simulink model "MSFartoystyring22"  (R2017b)
settings: Solver=ode45  StartTime=tstart  StopTime=tstop  RelTol=1e-3  EnableMultiTasking=on
values from neighbouring files (symbols this model uses):
  c = 1    [run22.m]
  p0 = [1500 500]    [run22.m]
  psi0 = 50*deg2rad    (= 0.872664625997)    [run22.m]
  r0 = 0    [run22.m]
  tsamp = 10    [run22.m]
  u_r_0 = v0(1)    [run22.m]
  v0 = [6.63 0]'    [run22.m]
undefined symbols (not defined in the file or in its folder): d1, d2, K, Kd_heading, Ki_heading, Ki_speed, Kp_heading, Kp_speed, m, msfartoystyring, omega_c, omega_n, T, WP, zeta_c
settings Model: ExtModeAutoUpdateStatusClock=off  Creator=christh  LastModifiedBy=henningward
settings SolverCC: ZeroCrossAlgorithm=Adaptive
settings DataIOCC: LimitDataPoints=on  SaveFormat=Array  SignalLoggingSaveFormat=ModelDataLogs
settings OptimizationCC: ExpressionDepthLimit=2147483647  InitFltsAndDblsToZero=on  LifeSpan=inf
settings DebuggingCC: UnderspecifiedInitializationDetection=Classic  MergeDetectMultiDrivingBlocksExec=none  IgnoredZcDiagnostic=none  SolverPrmCheckMsg=warning  FcnCallInpInsideContextMsg=warning  StateNameClashWarn=warning  SFUnexpectedBacktrackingDiag=warning  SFNoUnconditionalDefaultTransitionDiag=warning  SFExecutionAtInitializationDiag=none
settings HardwareCC: ProdBitPerPointer=32  ProdBitPerSizeT=32  ProdBitPerPtrDiffT=32  ProdLargestAtomicFloat=None  ProdIntDivRoundTo=Undefined  ProdEndianess=Unspecified  ProdWordSize=32  ProdHWDeviceType=32-bit Generic
settings ModelReferenceCC: PropagateSignalLabelsOutOfModel=off
settings CodeAppCC: StateflowObjectComments=on
settings GRTTargetCC: TargetLangStandard=C89/C90 (ANSI)  GeneratePreprocessorConditionals=Disable all  CombineOutputUpdateFcns=off  GRTInterface=on
settings ConfigComp: CovMetricSettings=dw  CovHtmlReporting=on  CovSaveCumulativeToWorkspaceVar=on  CovSaveSingleToWorkspaceVar=on  CovExternalEMLEnable=off

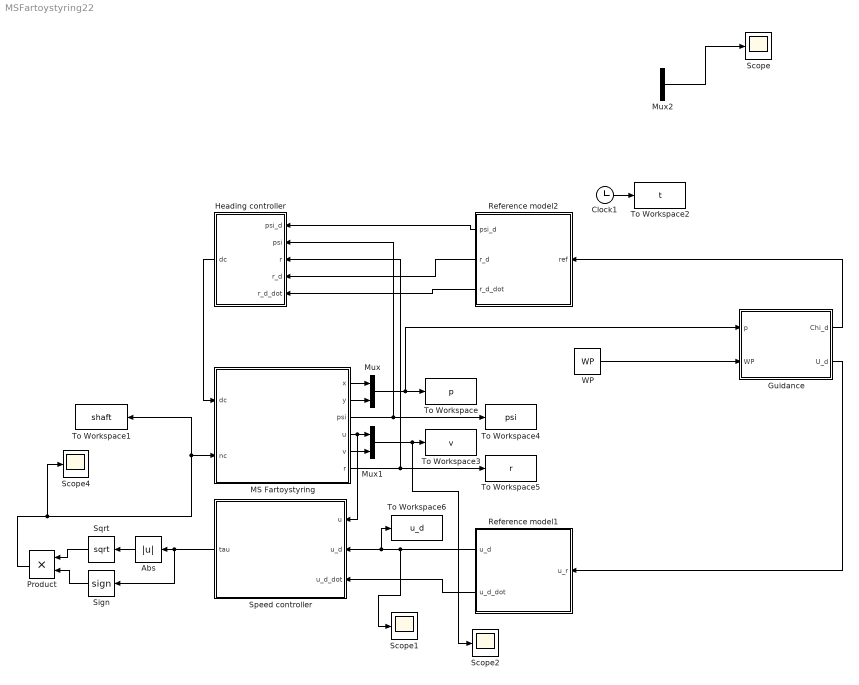
== system MSFartoystyring22 ==
  Abs : Abs
  Clock1 : Clock
  "Guidance " : Subsystem
  Heading controller : Subsystem
  MS Fartoystyring : Subsystem  mask(MS Fartoystyring for Assignment 3 G&C){x0=p0(1), y0=p0(2), u0=v0(1), v0=v0(2), psi0=psi0, r0=r0, c=c}
      mask prompts: x0 "x(t0) (m)"; y0 "y(t0) (m)"; u0 "u(t0) (m/s)"; v0 "v(t0) (m/s)"; psi0 "psi(t0) (rad)"; r0 "r(t0) (rad/s)"; c "current (0 or 1)"
      mask help:
      | Block corresponding to Figure 1 in the assignment text. Gives the response of the ship.
      |
      | The design speed of MS Fartoystyring is u=8.23 m/s.
      |
      | Input:
      | dc: commanded rudder (rad), dmax=25*pi/180
      | nc: commanded shaft speed (rad/s), nmax=85*2*pi/60
      |
      | Output:
      | x: north pos (m)
      | y: east pos (m)
      | u: surge (m/s)
      | v: sway (m/s)
      | psi: heading (rad)
      | r: yaw (rad/s)
      mask Help: Comments, bugs and help requests can be directed to the TA. Email on course website.
  Mux : Mux  Inputs=2
  Mux1 : Mux  Inputs=2
  Mux2 : Mux  Inputs=2
  Product : Product
  Reference model1 : Subsystem
  Reference model2 : Subsystem
  Scope{,1..2,4} (4 alike) : Scope
  Sign : Signum
  Speed controller : Subsystem
  Sqrt : Sqrt  SaturateOnIntegerOverflow=on
  To Workspace : ToWorkspace  VariableName=p  SampleTime=tsamp
  To Workspace1 : ToWorkspace  VariableName=shaft  SampleTime=tsamp
  To Workspace2 : ToWorkspace  VariableName=t  SampleTime=tsamp
  To Workspace3 : ToWorkspace  VariableName=v  SampleTime=tsamp
  To Workspace4 : ToWorkspace  VariableName=psi  SampleTime=tsamp
  To Workspace5 : ToWorkspace  VariableName=r  SampleTime=tsamp
  To Workspace6 : ToWorkspace  VariableName=u_d  SampleTime=tsamp
  WP : Constant  Value=WP
  wires:
  MS Fartoystyring/1(x) -> Mux/1
  MS Fartoystyring/2(y) -> Mux/2
  MS Fartoystyring/4(u) -> Speed controller/1("u "), Mux1/1
  MS Fartoystyring/5(v) -> Mux1/2
  Mux/1 -> "Guidance "/1(p), To Workspace/1
  Clock1/1 -> To Workspace2/1
  Speed controller/1("tau ") -> Sign/1, Abs/1
  Abs/1 -> Sqrt/1
  Sign/1 -> Product/2
  Sqrt/1 -> Product/1
  Product/1 -> Scope4/1, To Workspace1/1, MS Fartoystyring/2(nc)
  Reference model1/1(u_d) -> Scope1/1, To Workspace6/1, Speed controller/2(u_d)
  Reference model1/2(u_d_dot) -> Speed controller/3(u_d_dot)
  WP/1 -> "Guidance "/2(WP)
  Reference model2/2(r_d) -> Heading controller/4(r_d)
  MS Fartoystyring/6(r) -> Heading controller/3(r), To Workspace5/1
  MS Fartoystyring/3(psi) -> Heading controller/2(psi), To Workspace4/1
  Reference model2/3("r_d_dot ") -> Heading controller/5("r_d_dot ")
  Mux1/1 -> Scope2/1, To Workspace3/1
  Heading controller/1(dc) -> MS Fartoystyring/1(dc)
  Reference model2/1(psi_d) -> Heading controller/1(psi_d)
  Mux2/1 -> Scope/1
  "Guidance "/1("Chi_d ") -> Reference model2/1(ref)
  "Guidance "/2(U_d) -> Reference model1/1(u_r)

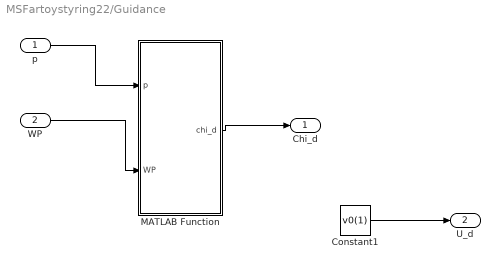
== system MSFartoystyring22/Guidance  ==
  p : Inport
  WP : Inport  Port=2
  Constant1 : Constant  Value=v0(1)
  MATLAB Function : MATLAB Function  TreatAsAtomicUnit=on
  "Chi_d " : Outport
  U_d : Outport  Port=2
  wires:
  p/1 -> MATLAB Function/1(p)
  WP/1 -> MATLAB Function/2(WP)
  Constant1/1 -> U_d/1
  MATLAB Function/1(chi_d) -> "Chi_d "/1

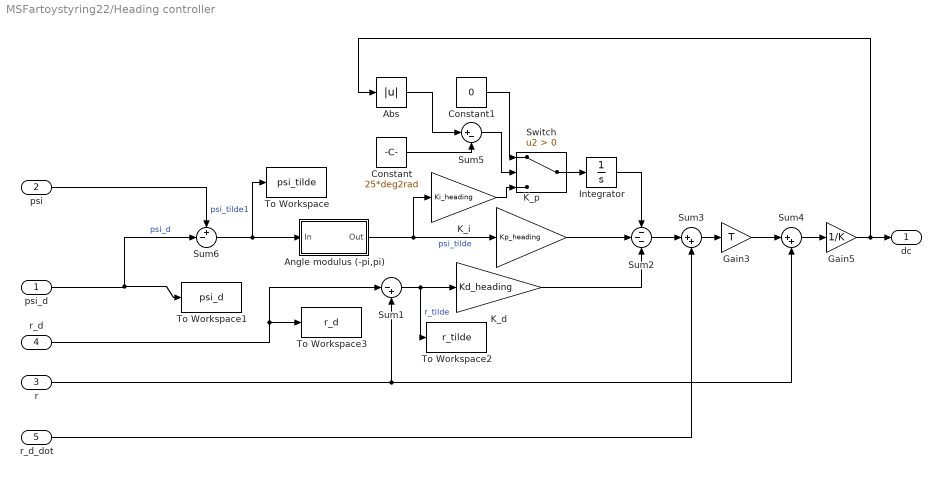
== system MSFartoystyring22/Heading controller ==
  psi_d : Inport
  psi : Inport  Port=2
  r : Inport  Port=3
  r_d : Inport  Port=4
  "r_d_dot " : Inport  Port=5
  Abs : Abs
  Angle modulus (-pi,pi) : Subsystem
  Constant : Constant  Value=25*deg2rad
  Constant1 : Constant  Value=0
  Gain3 : Gain  Gain=T
  Gain5 : Gain  Gain=1/K
  Integrator : Integrator  LimitOutput=on  UpperSaturationLimit=deg2rad*25*abs(K)/T  LowerSaturationLimit=-deg2rad*25*abs(K)/T
  K_d : Gain  Gain=Kd_heading
  K_i : Gain  Gain=Ki_heading
  K_p : Gain  Gain=Kp_heading
  Sum1 : Sum  Inputs=|-+
  Sum2 : Sum  Inputs=---
  Sum3 : Sum  Inputs=|++
  Sum4 : Sum  Inputs=|++
  Sum5 : Sum  Inputs=|+-
  Sum6 : Sum  Inputs=+-|
  Switch : Switch  Criteria=u2 > Threshold
  To Workspace : ToWorkspace  VariableName=psi_tilde  SampleTime=tsamp
  To Workspace1 : ToWorkspace  VariableName=psi_d  SampleTime=tsamp
  To Workspace2 : ToWorkspace  VariableName=r_tilde  SampleTime=tsamp
  To Workspace3 : ToWorkspace  VariableName=r_d  SampleTime=tsamp
  dc : Outport
  wires:
  Sum1/1 -> To Workspace2/1, K_d/1  "r_tilde"
  Angle modulus (-pi,pi)/1(Out) -> K_p/1, K_i/1  "psi_tilde"
  K_p/1 -> Sum2/2
  Sum2/1 -> Sum3/1
  K_d/1 -> Sum2/3
  Sum3/1 -> Gain3/1
  Gain3/1 -> Sum4/1
  r/1 -> Sum4/2, Sum1/2
  Gain5/1 -> Abs/1, dc/1
  Sum4/1 -> Gain5/1
  Integrator/1 -> Sum2/1
  Abs/1 -> Sum5/1
  Sum5/1 -> Switch/2
  Constant/1 -> Sum5/2
  Constant1/1 -> Switch/1
  K_i/1 -> Switch/3
  Switch/1 -> Integrator/1
  psi_d/1 -> To Workspace1/1, Sum6/2  "psi_d"
  Sum6/1 -> To Workspace/1, Angle modulus (-pi,pi)/1(In)  "psi_tilde1"
  psi/1 -> Sum6/1
  "r_d_dot "/1 -> Sum3/2
  r_d/1 -> To Workspace3/1, Sum1/1

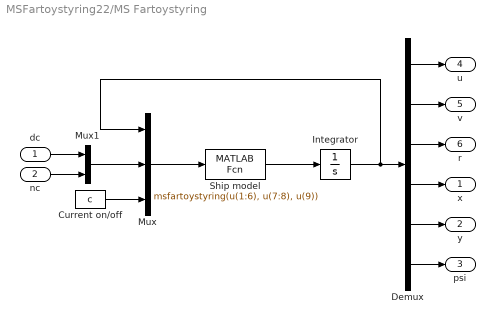
== system MSFartoystyring22/MS Fartoystyring ==
  dc : Inport
  nc : Inport  Port=2
  Current on/off : Constant  Value=c
  Demux : Demux  Outputs=6
  Integrator : Integrator  InitialCondition=[u0 v0 r0 x0 y0 psi0]'
  Mux : Mux  Inputs=3
  Mux1 : Mux  Inputs=2
  Ship model : MATLABFcn  MATLABFcn=msfartoystyring(u(1:6), u(7:8), u(9))  OutputDimensions=6
  x : Outport
  y : Outport  Port=2
  psi : Outport  Port=3
  u : Outport  Port=4
  v : Outport  Port=5
  r : Outport  Port=6
  wires:
  Integrator/1 -> Mux/1, Demux/1
  Mux1/1 -> Mux/2
  dc/1 -> Mux1/1
  nc/1 -> Mux1/2
  Demux/1 -> u/1
  Demux/2 -> v/1
  Demux/3 -> r/1
  Demux/4 -> x/1
  Demux/5 -> y/1
  Demux/6 -> psi/1
  Current on/off/1 -> Mux/3
  Ship model/1 -> Integrator/1
  Mux/1 -> Ship model/1

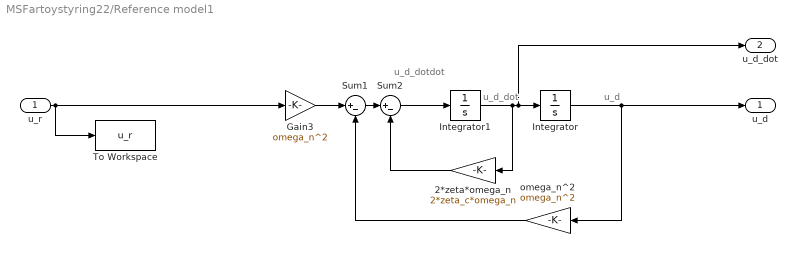
== system MSFartoystyring22/Reference model1 ==
  note: u_d
  note: u_d_dot
  note: u_d_dotdot
  u_r : Inport
  2*zeta*omega_n : Gain  Gain=2*zeta_c*omega_n
  Gain3 : Gain  Gain=omega_n^2
  Integrator : Integrator  InitialCondition=u_r_0
  Integrator1 : Integrator
  Sum1 : Sum  Inputs=|+-
  Sum2 : Sum  Inputs=|+-
  To Workspace : ToWorkspace  VariableName=u_r  SampleTime=-1
  omega_n^2 : Gain  Gain=omega_n^2
  u_d : Outport
  u_d_dot : Outport  Port=2
  wires:
  Integrator1/1 -> 2*zeta*omega_n/1, Integrator/1, u_d_dot/1
  2*zeta*omega_n/1 -> Sum2/2
  Sum1/1 -> Sum2/1
  omega_n^2/1 -> Sum1/2
  Gain3/1 -> Sum1/1
  Sum2/1 -> Integrator1/1
  Integrator/1 -> omega_n^2/1, u_d/1
  u_r/1 -> To Workspace/1, Gain3/1

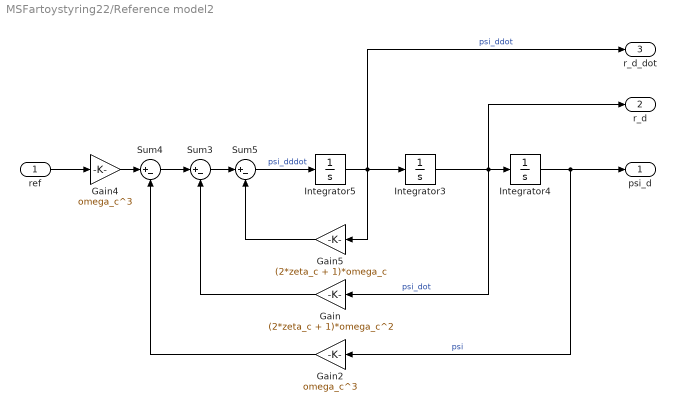
== system MSFartoystyring22/Reference model2 ==
  ref : Inport
  Gain : Gain  Gain=(2*zeta_c + 1)*omega_c^2
  Gain2 : Gain  Gain=omega_c^3
  Gain4 : Gain  Gain=omega_c^3
  Gain5 : Gain  Gain=(2*zeta_c + 1)*omega_c
  Integrator3 : Integrator
  Integrator4 : Integrator  InitialCondition=psi0
  Integrator5 : Integrator
  Sum3 : Sum  Inputs=|+-
  Sum4 : Sum  Inputs=|+-
  Sum5 : Sum  Inputs=|+-
  psi_d : Outport
  r_d : Outport  Port=2
  "r_d_dot " : Outport  Port=3
  wires:
  Integrator3/1 -> r_d/1, Gain/1, Integrator4/1  "psi_dot"
  Gain/1 -> Sum3/2
  ref/1 -> Gain4/1
  Integrator4/1 -> psi_d/1, Gain2/1  "psi"
  Sum4/1 -> Sum3/1
  Gain4/1 -> Sum4/1
  Sum3/1 -> Sum5/1
  Gain5/1 -> Sum5/2
  Sum5/1 -> Integrator5/1  "psi_dddot"
  Gain2/1 -> Sum4/2
  Integrator5/1 -> Gain5/1, "r_d_dot "/1, Integrator3/1  "psi_ddot"

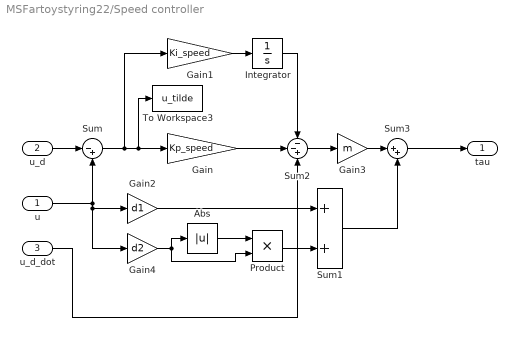
== system MSFartoystyring22/Speed controller ==
  "u " : Inport
  u_d : Inport  Port=2
  u_d_dot : Inport  Port=3
  Abs : Abs
  Gain : Gain  Gain=Kp_speed
  Gain1 : Gain  Gain=Ki_speed
  Gain2 : Gain  Gain=d1
  Gain3 : Gain  Gain=m
  Gain4 : Gain  Gain=d2
  Integrator : Integrator
  Product : Product
  Sum : Sum  Inputs=|-+
  Sum1 : Sum
  Sum2 : Sum  Inputs=--+
  Sum3 : Sum  Inputs=|++
  To Workspace3 : ToWorkspace  VariableName=u_tilde  SampleTime=tsamp
  "tau " : Outport
  wires:
  Integrator/1 -> Sum2/1
  Gain/1 -> Sum2/2
  Sum2/1 -> Gain3/1
  Gain3/1 -> Sum3/1
  u_d_dot/1 -> Sum2/3
  Sum/1 -> To Workspace3/1, Gain/1, Gain1/1
  Gain1/1 -> Integrator/1
  u_d/1 -> Sum/1
  "u "/1 -> Gain4/1, Gain2/1, Sum/2
  Abs/1 -> Product/1
  Gain4/1 -> Abs/1, Product/2
  Gain2/1 -> Sum1/1
  Product/1 -> Sum1/2
  Sum1/1 -> Sum3/2
  Sum3/1 -> "tau "/1

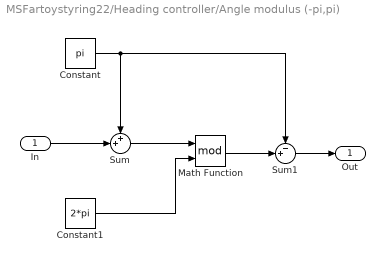
== system MSFartoystyring22/Heading controller/Angle modulus (-pi,pi) ==
  In : Inport
  Constant : Constant  Value=pi
  Constant1 : Constant  Value=2*pi
  Math Function : Math  Operator=mod  SaturateOnIntegerOverflow=on
  Sum : Sum  Inputs=++|
  Sum1 : Sum  Inputs=-+|
  Out : Outport
  wires:
  Math Function/1 -> Sum1/2
  Sum/1 -> Math Function/1
  Constant/1 -> Sum1/1, Sum/1
  In/1 -> Sum/2
  Sum1/1 -> Out/1
  Constant1/1 -> Math Function/2

== matlab function MSFartoystyring22/Guidance /MATLAB Function ==
  settings: updateMethod=DISCRETE  sampleTime=tsamp
  data: p input; chi_d output; WP input
function chi_d = fcn(p, WP)

    %number of waypoints
    N = length(WP);

    % waypoint iteration
    persistent k;
    
    %waypoint iteration
    if (isempty(k))
        k = 1;
    end
    
    %reference waypoint
    xk_ref = WP(1, k);
    yk_ref = WP(2, k);
    
    %next waypoint
    xk_target = WP(1, k+1);
    yk_target = WP(2, k+1);
    
    
    if k ~= 6 && k ~= 1
        %calculating optimal turningradius
        lastWP = [WP(1,k-1); WP(2,k-1)];
        currentWP = [WP(1,k); WP(2,k)]; %way points
        nextWP = [WP(1,k+1); WP(2,k+1)];
        u = (lastWP - currentWP)/(norm(lastWP-currentWP));
        v = (nextWP - currentWP)/(norm(nextWP-currentWP)); %a,b,c
        w = (u + v)/(norm(u) + norm(v));
        a = acos((norm(v)^2 + norm(u+v)^2 - norm(u)^2)/(2*norm(v)*norm(u+v)));
        turningRadius = 900 / sin(a)*1.3;
    else
        turningRadius = 900*1.3;
    end
    
   
    alpha_k = atan2(yk_target-yk_ref, xk_target-xk_ref);
    
    Rp = [cos(alpha_k) -sin(alpha_k);
          sin(alpha_k) cos(alpha_k);];
      
    epsilon = Rp'*(p - [xk_ref yk_ref]');
    
    %R = sqrt(((xk_target-xk_ref)^2+(yk_target-yk_ref)^2))-epsilon(1,:); %Radius of acceptance
    chi_p = alpha_k;
    s = epsilon(1);
    e = epsilon(2);
    
    %{
    if ((((xk_ref - p(1))^2 + (yk_ref - p(2))^2) <= 900^2) && (N > k))
        k = k + 1;
    end   
    %}
    
    Delta = 600;
    
    chi_r = atan(-e/Delta);
    chi_d = chi_p+chi_r;
    chi_d = mod(chi_d, 2*pi);
    
    
    if (norm(WP(:, k+1)-WP(:, k)) - s <= turningRadius) && (N-1 > k)
       k = k + 1;
    end
    
    
    
    
    
 
    
end
